simulink model "EGRVlv_VDMon"  (R2018a)
settings: configuration reference "cs_ert" (kept outside this file)
model workspace (MAT data in the model file):
  EGRVlv_VDMon_DT = 10
values from neighbouring files (symbols this model uses):
  EGRVlv_drActDvt_C = 2.0    [EGRVlv_VDMon.sldd]
  EGRVlv_drActDvtHi_C = 4.0    [EGRVlv_VDMon.sldd]
  EGRVlv_numJamVlv_C = 2.0    [EGRVlv_VDMon.sldd]
  EGRVlv_numLckdDetThres_C = 0.0    [EGRVlv_VDMon.sldd]
  EGRVlv_numMonEngTemp_C = 0.0    [EGRVlv_VDMon.sldd]
  EGRVlv_rDvtMax_C = 10.0    [EGRVlv_VDMon.sldd]
  EGRVlv_rDvtMin_C = 5.0    [EGRVlv_VDMon.sldd]
  EGRVlv_rLckdDetThres_C = 5.0    [EGRVlv_VDMon.sldd]
  EGRVlv_rLMSActPosThresInit_C = 3.0    [EGRVlv_VDMon.sldd]
  EGRVlv_rLMSActThresDwn_C = 5.0    [EGRVlv_VDMon.sldd]
  EGRVlv_rLMSThresDwn_C = 5.0    [EGRVlv_VDMon.sldd]
  EGRVlv_rLMSThresUp_C = 10.0    [EGRVlv_VDMon.sldd]
  EGRVlv_RlsIKi_C = 5.0    [EGRVlv_VDMon.sldd]
  EGRVlv_rRlsMax_C = 80.0    [EGRVlv_VDMon.sldd]
  EGRVlv_rStpThres_C = 2.0    [EGRVlv_VDMon.sldd]
  EGRVlv_tEngHi_C = 200.0    [EGRVlv_VDMon.sldd]
  EGRVlv_tEngLo_C = 150.0    [EGRVlv_VDMon.sldd]
  EGRVlv_tiGovDvtMaxDebDef_C = 200.0    [EGRVlv_VDMon.sldd]
  EGRVlv_tiGovDvtMaxDebOk_C = 200.0    [EGRVlv_VDMon.sldd]
  EGRVlv_tiGovDvtMinDebDef_C = 200.0    [EGRVlv_VDMon.sldd]
  EGRVlv_tiGovDvtMinDebOk_C = 200.0    [EGRVlv_VDMon.sldd]
  EGRVlv_tiLMS_C = 1.0    [EGRVlv_VDMon.sldd]
  EGRVlv_tiRepRls_C = 1.0    [EGRVlv_VDMon.sldd]
  EGRVlv_tiRls_C = 1.0    [EGRVlv_VDMon.sldd]
undefined symbols (not defined in the file or in its folder): EngState
libraries: simulink x25, sllib x6
settings Model: DataDictionary=EGRVlv_VDMon.sldd  Creator=zhoutinglin  LastModifiedBy=zhoutinglin

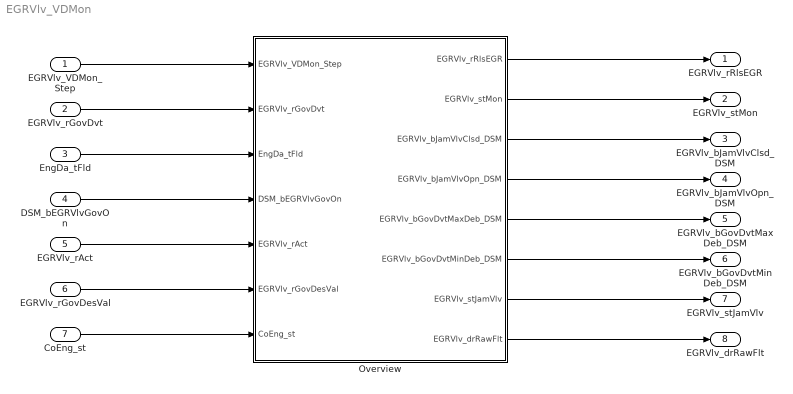
== system EGRVlv_VDMon ==
  EGRVlv_VDMon_Step : Inport  OutputFunctionCall=on
  EGRVlv_rGovDvt : Inport  Description=Control deviation  Port=2  OutMin=-100  OutMax=100  OutDataTypeStr=DutyCycle  Unit=%  PortDimensions=[1 1]
  EngDa_tFld : Inport  Description=Engine temperature field  Port=3  OutMin=-3000  OutMax=3000  OutDataTypeStr=Temp_C  Unit=deg  PortDimensions=[1 3]
  DSM_bEGRVlvGovOn : Inport  Description=Status of FId_EGRVlvGovOn  Port=4  OutMin=0  OutMax=1  OutDataTypeStr=boolean  PortDimensions=[1 1]
  EGRVlv_rAct : Inport  Description=Actuatorposition  Port=5  OutMin=-100  OutMax=100  OutDataTypeStr=DutyCycle  Unit=%  PortDimensions=[1 1]
  EGRVlv_rGovDesVal : Inport  Description=Internal desired value for governor  Port=6  OutMin=-100  OutMax=100  OutDataTypeStr=DutyCycle  Unit=%  PortDimensions=[1 1]
  CoEng_st : Inport  Description=Engine coordinator state  Port=7  OutDataTypeStr=Enum:EngState  PortDimensions=[1 1]
  Overview : Subsystem
  EGRVlv_rRlsEGR : Outport  Description=Additional control value to release a jammed valve  OutMin=-100  OutMax=100  OutDataTypeStr=DutyCycle  Unit=%  PortDimensions=[1 1]
  EGRVlv_stMon : Outport  Description=State of system monitoring  Port=2  OutMin=0  OutMax=65535  OutDataTypeStr=State2  PortDimensions=[1 1]
  EGRVlv_bJamVlvClsd_DSM : Outport  Description=Status of EGRVlv_bJamVlvClsd  Port=3  OutMin=0  OutMax=1  OutDataTypeStr=boolean  PortDimensions=[1 1]
  EGRVlv_bJamVlvOpn_DSM : Outport  Description=Status of EGRVlv_bJamVlvOpn  Port=4  OutMin=0  OutMax=1  OutDataTypeStr=boolean  PortDimensions=[1 1]
  EGRVlv_bGovDvtMaxDeb_DSM : Outport  Description=Status of EGRVlv_bGovDvtMaxDeb  Port=5  OutMin=0  OutMax=1  OutDataTypeStr=boolean  PortDimensions=[1 1]
  EGRVlv_bGovDvtMinDeb_DSM : Outport  Description=Status of EGRVlv_bGovDvtMinDeb  Port=6  OutMin=0  OutMax=1  OutDataTypeStr=boolean  PortDimensions=[1 1]
  EGRVlv_stJamVlv : Outport  Description=Status indicates that the valve is jammed  Port=7  OutMin=0  OutMax=1  OutDataTypeStr=boolean  PortDimensions=[1 1]
  EGRVlv_drRawFlt : Outport  Description=EGR rate gradient calculated over current position after PT1-filtering  Port=8  OutMin=-100  OutMax=100  OutDataTypeStr=DutyCycle  Unit=r/s  PortDimensions=[1 1]
  wires:
  EGRVlv_VDMon_Step/1 -> Overview/1(EGRVlv_VDMon_Step)
  EGRVlv_rGovDvt/1 -> Overview/2(EGRVlv_rGovDvt)
  EngDa_tFld/1 -> Overview/3(EngDa_tFld)
  DSM_bEGRVlvGovOn/1 -> Overview/4(DSM_bEGRVlvGovOn)
  EGRVlv_rAct/1 -> Overview/5(EGRVlv_rAct)
  EGRVlv_rGovDesVal/1 -> Overview/6(EGRVlv_rGovDesVal)
  CoEng_st/1 -> Overview/7(CoEng_st)
  Overview/1(EGRVlv_rRlsEGR) -> EGRVlv_rRlsEGR/1
  Overview/2(EGRVlv_stMon) -> EGRVlv_stMon/1
  Overview/3(EGRVlv_bJamVlvClsd_DSM) -> EGRVlv_bJamVlvClsd_DSM/1
  Overview/4(EGRVlv_bJamVlvOpn_DSM) -> EGRVlv_bJamVlvOpn_DSM/1
  Overview/5(EGRVlv_bGovDvtMaxDeb_DSM) -> EGRVlv_bGovDvtMaxDeb_DSM/1
  Overview/6(EGRVlv_bGovDvtMinDeb_DSM) -> EGRVlv_bGovDvtMinDeb_DSM/1
  Overview/7(EGRVlv_stJamVlv) -> EGRVlv_stJamVlv/1
  Overview/8(EGRVlv_drRawFlt) -> EGRVlv_drRawFlt/1

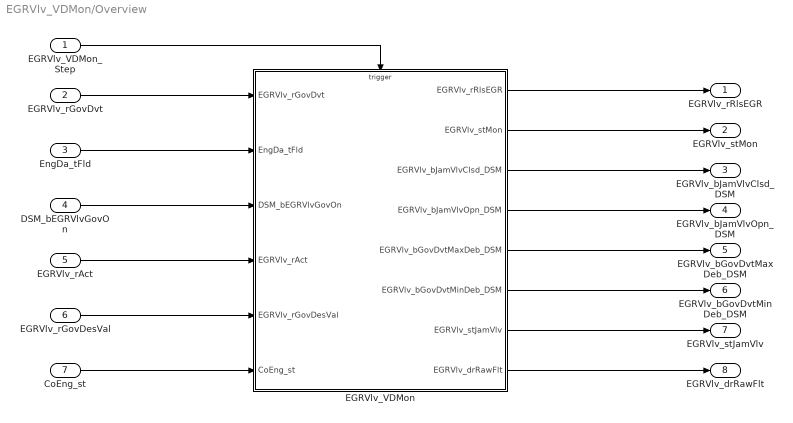
== system EGRVlv_VDMon/Overview ==
  EGRVlv_VDMon_Step : Inport
  EGRVlv_rGovDvt : Inport  Port=2
  EngDa_tFld : Inport  Port=3
  DSM_bEGRVlvGovOn : Inport  Port=4
  EGRVlv_rAct : Inport  Port=5
  EGRVlv_rGovDesVal : Inport  Port=6
  CoEng_st : Inport  Port=7
  EGRVlv_VDMon : Subsystem
  EGRVlv_rRlsEGR : Outport
  EGRVlv_stMon : Outport  Port=2
  EGRVlv_bJamVlvClsd_DSM : Outport  Port=3
  EGRVlv_bJamVlvOpn_DSM : Outport  Port=4
  EGRVlv_bGovDvtMaxDeb_DSM : Outport  Port=5
  EGRVlv_bGovDvtMinDeb_DSM : Outport  Port=6
  EGRVlv_stJamVlv : Outport  Port=7
  EGRVlv_drRawFlt : Outport  Port=8
  wires:
  EGRVlv_rGovDvt/1 -> EGRVlv_VDMon/1(EGRVlv_rGovDvt)
  EngDa_tFld/1 -> EGRVlv_VDMon/2(EngDa_tFld)
  DSM_bEGRVlvGovOn/1 -> EGRVlv_VDMon/3(DSM_bEGRVlvGovOn)
  EGRVlv_rAct/1 -> EGRVlv_VDMon/4(EGRVlv_rAct)
  EGRVlv_rGovDesVal/1 -> EGRVlv_VDMon/5(EGRVlv_rGovDesVal)
  CoEng_st/1 -> EGRVlv_VDMon/6(CoEng_st)
  EGRVlv_VDMon/1(EGRVlv_rRlsEGR) -> EGRVlv_rRlsEGR/1
  EGRVlv_VDMon/2(EGRVlv_stMon) -> EGRVlv_stMon/1
  EGRVlv_VDMon/3(EGRVlv_bJamVlvClsd_DSM) -> EGRVlv_bJamVlvClsd_DSM/1
  EGRVlv_VDMon/4(EGRVlv_bJamVlvOpn_DSM) -> EGRVlv_bJamVlvOpn_DSM/1
  EGRVlv_VDMon/5(EGRVlv_bGovDvtMaxDeb_DSM) -> EGRVlv_bGovDvtMaxDeb_DSM/1
  EGRVlv_VDMon/6(EGRVlv_bGovDvtMinDeb_DSM) -> EGRVlv_bGovDvtMinDeb_DSM/1
  EGRVlv_VDMon/7(EGRVlv_stJamVlv) -> EGRVlv_stJamVlv/1
  EGRVlv_VDMon/8(EGRVlv_drRawFlt) -> EGRVlv_drRawFlt/1
  EGRVlv_VDMon_Step/1 -> EGRVlv_VDMon/Trigger

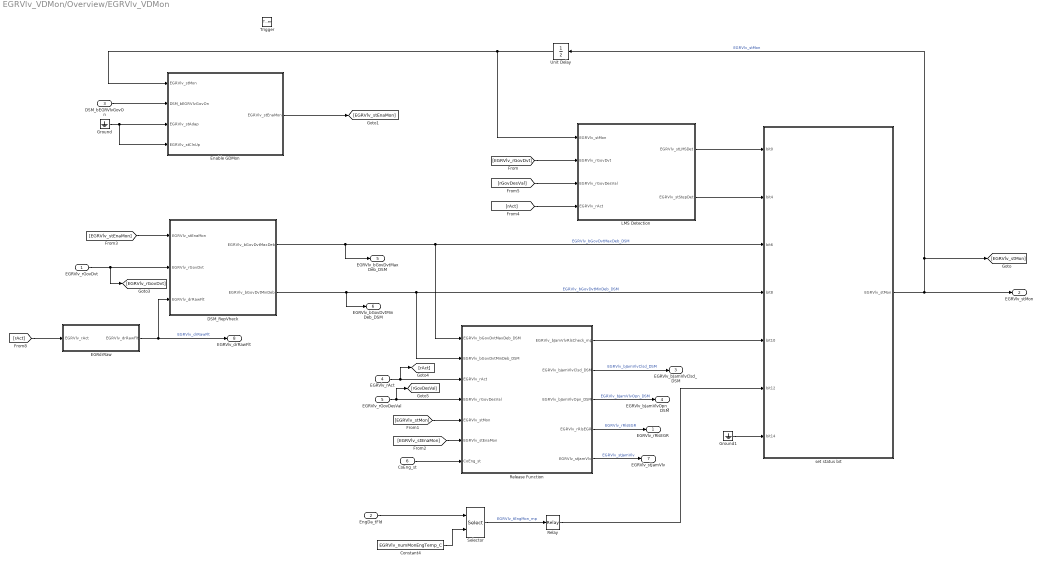
== system EGRVlv_VDMon/Overview/EGRVlv_VDMon ==
  EGRVlv_rGovDvt : Inport  Tag=%
  EngDa_tFld : Inport  Tag=%  Port=2
  DSM_bEGRVlvGovOn : Inport  Tag=%  Port=3
  EGRVlv_rAct : Inport  Tag=%  Port=4
  EGRVlv_rGovDesVal : Inport  Tag=%  Port=5
  CoEng_st : Inport  Tag=%  Port=6
  Trigger : TriggerPort  TriggerType=function-call  VariantControl=Variant  PortDimensions=1
  Constant4 : Constant  Value=EGRVlv_numMonEngTemp_C  SampleTime=-1
  DSM_RepVheck : Subsystem
  EGRdrRaw : Subsystem
  Enable GDMon : Subsystem
  Ground : Ground
  Ground1 : Ground
  LMS Detection : Subsystem
  Relay : Relay  OnSwitchValue=EGRVlv_tEngHi_C  OffSwitchValue=EGRVlv_tEngLo_C
  Release Function : Subsystem
  Selector : Selector  IndexMode=Zero-based  InputPortWidth=3  IndexOptions=Index vector (port)  Indices=[1 3]  OutputSizes=1
  Unit Delay : UnitDelay  SampleTime=-1
      settings: AttributesFormatString=InitialValue=%<InitialCondition>
  set status bit : Subsystem
  EGRVlv_rRlsEGR : Outport  Tag=%
  EGRVlv_stMon : Outport  Tag=%  Port=2
  EGRVlv_bJamVlvClsd_DSM : Outport  Tag=%  Port=3
  EGRVlv_bJamVlvOpn_DSM : Outport  Tag=%  Port=4
  EGRVlv_bGovDvtMaxDeb_DSM : Outport  Port=5
  EGRVlv_bGovDvtMinDeb_DSM : Outport  Port=6
  EGRVlv_stJamVlv : Outport  Port=7
  EGRVlv_drRawFlt : Outport  Port=8
  wires:
  Selector/1 -> Relay/1  "EGRVlv_tEngMon_mp"
  set status bit/1(EGRVlv_stMon) -> EGRVlv_stMon/1, Unit Delay/1, [EGRVlv_stMon]  "EGRVlv_stMon"
  Constant4/1 -> Selector/2
  EngDa_tFld/1 -> Selector/1
  EGRVlv_rGovDvt/1 -> [EGRVlv_rGovDvt], DSM_RepVheck/2(EGRVlv_rGovDvt)
  EGRVlv_rAct/1 -> [rAct], Release Function/3(EGRVlv_rAct)
  EGRVlv_rGovDesVal/1 -> [rGovDesVal], Release Function/4(EGRVlv_rGovDesVal)
  Unit Delay/1 -> Enable GDMon/1(EGRVlv_stMon), LMS Detection/1(EGRVlv_stMon)
  LMS Detection/2(EGRVlv_stStepDet) -> set status bit/2(bit4)
  LMS Detection/1(EGRVlv_stLMSDet) -> set status bit/1(bit0)
  Enable GDMon/1(EGRVlv_stEnaMon) -> [EGRVlv_stEnaMon]
  DSM_bEGRVlvGovOn/1 -> Enable GDMon/2(DSM_bEGRVlvGovOn)
  Ground/1 -> Enable GDMon/4(EGRVlv_stClnUp), Enable GDMon/3(EGRVlv_stAdap)
  [EGRVlv_rGovDvt] -> LMS Detection/2(EGRVlv_rGovDvt)
  [rGovDesVal] -> LMS Detection/3(EGRVlv_rGovDesVal)
  [rAct] -> LMS Detection/4(EGRVlv_rAct)
  [EGRVlv_stMon] -> Release Function/5(EGRVlv_stMon)
  [EGRVlv_stEnaMon] -> Release Function/6(EGRVlv_stEnaMon)
  CoEng_st/1 -> Release Function/7(CoEng_st)
  Ground1/1 -> set status bit/7(bit14)
  Release Function/2(EGRVlv_bJamVlvClsd_DSM) -> EGRVlv_bJamVlvClsd_DSM/1  "EGRVlv_bJamVlvClsd_DSM"
  Release Function/3(EGRVlv_bJamVlvOpn_DSM) -> EGRVlv_bJamVlvOpn_DSM/1  "EGRVlv_bJamVlvOpn_DSM"
  Release Function/4(EGRVlv_rRlsEGR) -> EGRVlv_rRlsEGR/1  "EGRVlv_rRlsEGR"
  DSM_RepVheck/2(EGRVlv_bGovDvtMinDeb) -> Release Function/2(EGRVlv_bGovDvtMinDeb_DSM), set status bit/4(bit8), EGRVlv_bGovDvtMinDeb_DSM/1  "EGRVlv_bGovDvtMinDeb_DSM"
  DSM_RepVheck/1(EGRVlv_bGovDvtMaxDeb) -> set status bit/3(bit6), Release Function/1(EGRVlv_bGovDvtMaxDeb_DSM), EGRVlv_bGovDvtMaxDeb_DSM/1  "EGRVlv_bGovDvtMaxDeb_DSM"
  Relay/1 -> set status bit/6(bit12)
  Release Function/1(EGRVlv_bJamVlvRlsCheck_mp) -> set status bit/5(bit10)
  Release Function/5(EGRVlv_stJamVlv) -> EGRVlv_stJamVlv/1  "EGRVlv_stJamVlv"
  [rAct] -> EGRdrRaw/1(EGRVlv_rAct)
  EGRdrRaw/1(EGRVlv_drRawFlt) -> DSM_RepVheck/3(EGRVlv_drRawFlt), EGRVlv_drRawFlt/1  "EGRVlv_drRawFlt"
  [EGRVlv_stEnaMon] -> DSM_RepVheck/1(EGRVlv_stEnaMon)

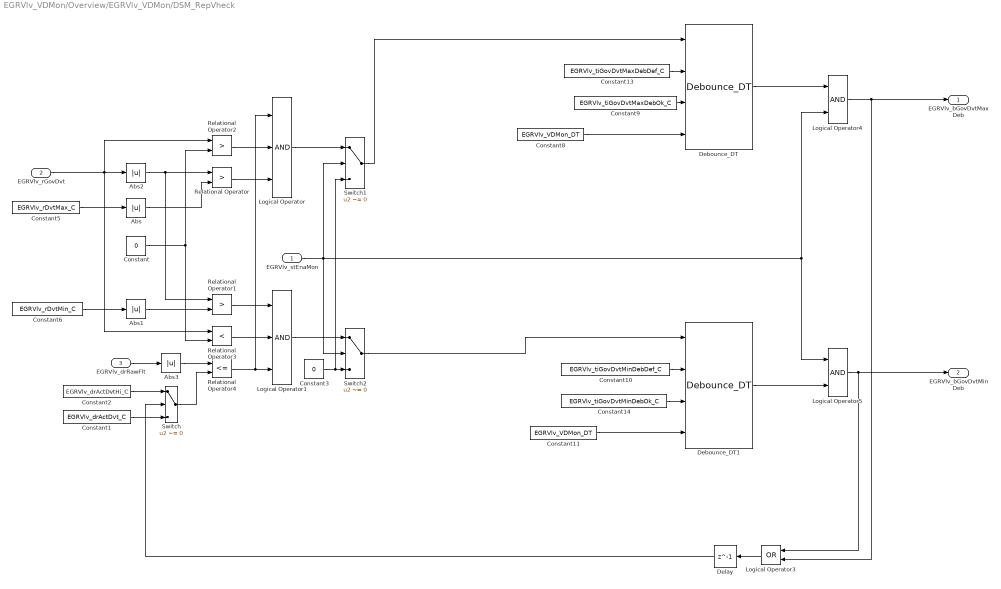
== system EGRVlv_VDMon/Overview/EGRVlv_VDMon/DSM_RepVheck ==
  EGRVlv_stEnaMon : Inport
  EGRVlv_rGovDvt : Inport  Tag=%  Port=2
  EGRVlv_drRawFlt : Inport  Port=3
  Abs{,1..3} (4 alike) : Abs
  Constant : Constant  Value=0  OutDataTypeStr=Inherit: Inherit via back propagation
  Constant1 : Constant  Value=EGRVlv_drActDvt_C  SampleTime=-1
  Constant10 : Constant  Value=EGRVlv_tiGovDvtMinDebDef_C
  Constant11 : Constant  Value=EGRVlv_VDMon_DT  OutDataTypeStr=Inherit: Inherit via back propagation
  Constant13 : Constant  Value=EGRVlv_tiGovDvtMaxDebDef_C
  Constant14 : Constant  Value=EGRVlv_tiGovDvtMinDebOk_C
  Constant2 : Constant  Value=EGRVlv_drActDvtHi_C  SampleTime=-1
  Constant3 : Constant  Value=0  OutDataTypeStr=Inherit: Inherit via back propagation
  Constant5 : Constant  Value=EGRVlv_rDvtMax_C  SampleTime=-1
  Constant6 : Constant  Value=EGRVlv_rDvtMin_C  SampleTime=-1
  Constant8 : Constant  Value=EGRVlv_VDMon_DT  OutDataTypeStr=Inherit: Inherit via back propagation
  Constant9 : Constant  Value=EGRVlv_tiGovDvtMaxDebOk_C
  Debounce_DT : sllib/Debounce_DT
      settings: SourceProductName=sllib
  Debounce_DT1 : sllib/Debounce_DT
      settings: SourceProductName=sllib
  Delay : Delay  DelayLength=1  InitialCondition=0
  Logical Operator : Logic  Inputs=3  AllPortsSameDT=off  OutDataTypeStr=boolean
  Logical Operator1 : Logic  Inputs=3  AllPortsSameDT=off  OutDataTypeStr=boolean
  Logical Operator3 : Logic  Operator=OR  AllPortsSameDT=off  OutDataTypeStr=boolean
  Logical Operator4 : Logic  AllPortsSameDT=off  OutDataTypeStr=boolean
  Logical Operator5 : Logic  AllPortsSameDT=off  OutDataTypeStr=boolean
  Relational Operator : RelationalOperator  Operator=>  OutDataTypeStr=boolean  RndMeth=Simplest  InputSameDT=on
  Relational Operator1 : RelationalOperator  Operator=>  OutDataTypeStr=boolean  RndMeth=Simplest
  Relational Operator2 : RelationalOperator  Operator=>  OutDataTypeStr=boolean  RndMeth=Simplest  InputSameDT=on
  Relational Operator3 : RelationalOperator  Operator=<  OutDataTypeStr=boolean  RndMeth=Simplest
  Relational Operator4 : RelationalOperator  Operator=<=  OutDataTypeStr=boolean  RndMeth=Simplest
  Switch : Switch  Criteria=u2 ~= 0
  Switch1 : Switch  Criteria=u2 ~= 0
  Switch2 : Switch  Criteria=u2 ~= 0
  EGRVlv_bGovDvtMaxDeb : Outport  OutputWhenDisabled=reset  InitialOutput=0
  EGRVlv_bGovDvtMinDeb : Outport  Port=2  OutputWhenDisabled=reset  InitialOutput=0
  wires:
  Relational Operator1/1 -> Logical Operator1/1
  Constant5/1 -> Abs/1
  Relational Operator3/1 -> Logical Operator1/2
  Constant8/1 -> Debounce_DT/4
  Abs/1 -> Relational Operator/2
  Abs2/1 -> Relational Operator1/1, Relational Operator/1
  Abs3/1 -> Relational Operator4/1
  EGRVlv_drRawFlt/1 -> Abs3/1
  Constant11/1 -> Debounce_DT1/4
  EGRVlv_rGovDvt/1 -> Relational Operator3/1, Relational Operator2/1, Abs2/1
  Constant13/1 -> Debounce_DT/2
  Relational Operator4/1 -> Logical Operator/1, Logical Operator1/3
  Relational Operator/1 -> Logical Operator/3
  Relational Operator2/1 -> Logical Operator/2
  Constant/1 -> Relational Operator3/2, Relational Operator2/2
  Abs1/1 -> Relational Operator1/2
  Constant14/1 -> Debounce_DT1/3
  Constant6/1 -> Abs1/1
  Constant10/1 -> Debounce_DT1/2
  Logical Operator3/1 -> Delay/1
  Delay/1 -> Switch/2
  Constant1/1 -> Switch/3
  Constant2/1 -> Switch/1
  Switch/1 -> Relational Operator4/2
  Switch1/1 -> Debounce_DT/1
  Logical Operator/1 -> Switch1/1
  Switch2/1 -> Debounce_DT1/1
  Logical Operator1/1 -> Switch2/1
  EGRVlv_stEnaMon/1 -> Switch1/2, Logical Operator5/1, Logical Operator4/2, Switch2/2
  Constant3/1 -> Switch1/3, Switch2/3
  Logical Operator4/1 -> EGRVlv_bGovDvtMaxDeb/1, Logical Operator3/2
  Debounce_DT/1 -> Logical Operator4/1
  Logical Operator5/1 -> EGRVlv_bGovDvtMinDeb/1, Logical Operator3/1
  Debounce_DT1/1 -> Logical Operator5/2
  Constant9/1 -> Debounce_DT/3

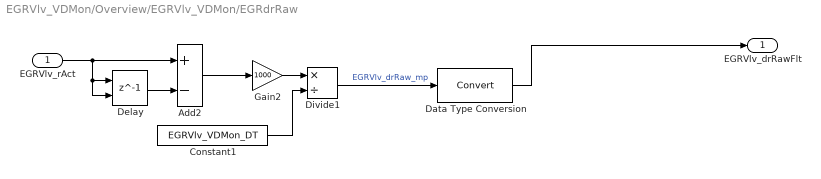
== system EGRVlv_VDMon/Overview/EGRVlv_VDMon/EGRdrRaw ==
  EGRVlv_rAct : Inport
  Add2 : Sum  Inputs=+-  SaturateOnIntegerOverflow=on
  Constant1 : Constant  Value=EGRVlv_VDMon_DT
  Data Type Conversion : DataTypeConversion
  Delay : Delay  DelayLength=1  InitialConditionSource=Input port  InitialCondition=0
      settings: InputPortMap=u0,p4
  Divide1 : Product  Inputs=*/  OutDataTypeStr=Inherit: Inherit via back propagation
  Gain2 : Gain  Gain=1000  OutDataTypeStr=fixdt(1,32,0.0001,0)  SaturateOnIntegerOverflow=on
  EGRVlv_drRawFlt : Outport
  wires:
  Delay/1 -> Add2/2
  EGRVlv_rAct/1 -> Delay/2, Delay/1, Add2/1
  Constant1/1 -> Divide1/2
  Gain2/1 -> Divide1/1
  Add2/1 -> Gain2/1
  Divide1/1 -> Data Type Conversion/1  "EGRVlv_drRaw_mp"
  Data Type Conversion/1 -> EGRVlv_drRawFlt/1

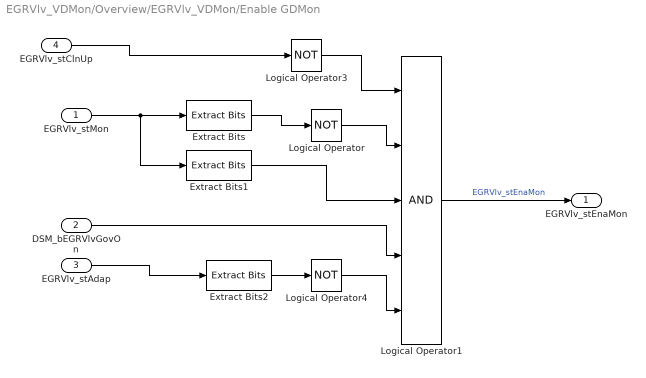
== system EGRVlv_VDMon/Overview/EGRVlv_VDMon/Enable GDMon ==
  EGRVlv_stMon : Inport  Tag=%
  DSM_bEGRVlvGovOn : Inport  Tag=%  Port=2
  EGRVlv_stAdap : Inport  Tag=%  Port=3
  EGRVlv_stClnUp : Inport  Tag=%  Port=4
  Extract Bits : simulink/Logic and Bit Operations/Extract Bits  bitsToExtract=Range of bits  numBits=8  bitIdxRange=[10 10]  outScalingMode=Treat bit field as an integer
      settings: SourceProductName=Simulink
  Extract Bits1 : simulink/Logic and Bit Operations/Extract Bits  bitsToExtract=Range of bits  numBits=8  bitIdxRange=[12 12]  outScalingMode=Treat bit field as an integer
      settings: SourceProductName=Simulink
  Extract Bits2 : simulink/Logic and Bit Operations/Extract Bits  bitsToExtract=Range of bits  numBits=8  bitIdxRange=[0 0]  outScalingMode=Treat bit field as an integer
      settings: SourceProductName=Simulink
  Logical Operator : Logic  Operator=NOT  AllPortsSameDT=off  OutDataTypeStr=boolean
  Logical Operator1 : Logic  Inputs=5  AllPortsSameDT=off  OutDataTypeStr=boolean
  Logical Operator3 : Logic  Operator=NOT  AllPortsSameDT=off  OutDataTypeStr=boolean
  Logical Operator4 : Logic  Operator=NOT  AllPortsSameDT=off  OutDataTypeStr=boolean
  EGRVlv_stEnaMon : Outport  Tag=%
  wires:
  Logical Operator/1 -> Logical Operator1/2
  Extract Bits1/1 -> Logical Operator1/3
  Extract Bits2/1 -> Logical Operator4/1
  EGRVlv_stClnUp/1 -> Logical Operator3/1
  Logical Operator4/1 -> Logical Operator1/5
  Logical Operator1/1 -> EGRVlv_stEnaMon/1  "EGRVlv_stEnaMon"
  DSM_bEGRVlvGovOn/1 -> Logical Operator1/4
  Extract Bits/1 -> Logical Operator/1
  EGRVlv_stMon/1 -> Extract Bits1/1, Extract Bits/1
  EGRVlv_stAdap/1 -> Extract Bits2/1
  Logical Operator3/1 -> Logical Operator1/1

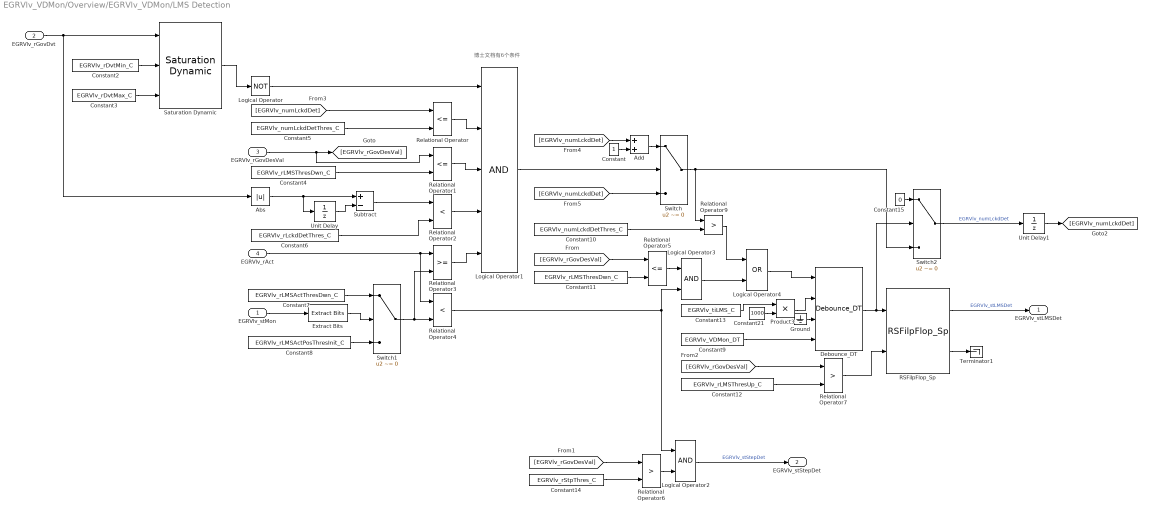
== system EGRVlv_VDMon/Overview/EGRVlv_VDMon/LMS Detection ==
  note: 博士文档有6个条件
  EGRVlv_stMon : Inport  Tag=%
  EGRVlv_rGovDvt : Inport  Tag=%  Port=2
  EGRVlv_rGovDesVal : Inport  Tag=%  Port=3
  EGRVlv_rAct : Inport  Tag=%  Port=4
  Abs : Abs
  Add : Sum  SaturateOnIntegerOverflow=on
  Constant : Constant  OutDataTypeStr=Inherit: Inherit via back propagation
  Constant10 : Constant  Value=EGRVlv_numLckdDetThres_C
  Constant11 : Constant  Value=EGRVlv_rLMSThresDwn_C
  Constant12 : Constant  Value=EGRVlv_rLMSThresUp_C
  Constant13 : Constant  Value=EGRVlv_tiLMS_C
  Constant14 : Constant  Value=EGRVlv_rStpThres_C
  Constant15 : Constant  Value=0  OutDataTypeStr=Inherit: Inherit via back propagation
  Constant2 : Constant  Value=EGRVlv_rDvtMin_C  SampleTime=-1
  Constant21 : Constant  Value=1000  OutDataTypeStr=uint16
  Constant3 : Constant  Value=EGRVlv_rDvtMax_C  SampleTime=-1
  Constant4 : Constant  Value=EGRVlv_rLMSThresDwn_C  SampleTime=-1
  Constant5 : Constant  Value=EGRVlv_numLckdDetThres_C  SampleTime=-1
  Constant6 : Constant  Value=EGRVlv_rLckdDetThres_C  SampleTime=-1
  Constant7 : Constant  Value=EGRVlv_rLMSActThresDwn_C  SampleTime=-1
  Constant8 : Constant  Value=EGRVlv_rLMSActPosThresInit_C  SampleTime=-1
  Constant9 : Constant  Value=EGRVlv_VDMon_DT
  Debounce_DT : sllib/Debounce_DT
      settings: SourceProductName=sllib
  Extract Bits : simulink/Logic and Bit Operations/Extract Bits  bitsToExtract=Range of bits  numBits=8  bitIdxRange=[14 14]  outScalingMode=Treat bit field as an integer
      settings: SourceProductName=Simulink
  Ground : Ground
  Logical Operator : Logic  Operator=NOT  AllPortsSameDT=off  OutDataTypeStr=boolean
  Logical Operator1 : Logic  Inputs=5  AllPortsSameDT=off  OutDataTypeStr=boolean
  Logical Operator2 : Logic  AllPortsSameDT=off  OutDataTypeStr=boolean
  Logical Operator3 : Logic  AllPortsSameDT=off  OutDataTypeStr=boolean
  Logical Operator4 : Logic  Operator=OR  AllPortsSameDT=off  OutDataTypeStr=boolean
  Product3 : Product  OutDataTypeStr=uint32  SaturateOnIntegerOverflow=on
  RSFilpFlop_Sp : sllib/RSFilpFlop_Sp
      settings: SourceProductName=sllib
  Relational Operator : RelationalOperator  Operator=<=  OutDataTypeStr=boolean  RndMeth=Simplest
  Relational Operator1 : RelationalOperator  Operator=<=  OutDataTypeStr=boolean  RndMeth=Simplest
  Relational Operator2 : RelationalOperator  Operator=<  OutDataTypeStr=boolean  RndMeth=Simplest
  Relational Operator3 : RelationalOperator  OutDataTypeStr=boolean  RndMeth=Simplest
  Relational Operator4 : RelationalOperator  Operator=<  OutDataTypeStr=boolean  RndMeth=Simplest
  Relational Operator5 : RelationalOperator  Operator=<=  OutDataTypeStr=boolean  RndMeth=Simplest
  Relational Operator6 : RelationalOperator  Operator=>  OutDataTypeStr=boolean  RndMeth=Simplest
  Relational Operator7 : RelationalOperator  Operator=>  OutDataTypeStr=boolean  RndMeth=Simplest
  Relational Operator9 : RelationalOperator  Operator=>  OutDataTypeStr=boolean  RndMeth=Simplest
  Saturation Dynamic : simulink/Discontinuities/Saturation Dynamic  OutMin=[]  OutMax=[]  OutDataTypeStr=Inherit: Same as second input  OutDataType=fixdt(1, 16)  OutScaling=2^-10  DoSatur=off
  Subtract : Sum  Inputs=+-  SaturateOnIntegerOverflow=on
  Switch : Switch  Criteria=u2 ~= 0
  Switch1 : Switch  Criteria=u2 ~= 0
  Switch2 : Switch  Criteria=u2 ~= 0
  Terminator1 : Terminator
  Unit Delay : UnitDelay  SampleTime=-1
      settings: AttributesFormatString=InitialValue=%<InitialCondition>
  Unit Delay1 : UnitDelay  SampleTime=-1
      settings: AttributesFormatString=InitialValue=%<InitialCondition>
  EGRVlv_stLMSDet : Outport  Tag=%
  EGRVlv_stStepDet : Outport  Tag=%  Port=2
  wires:
  Saturation Dynamic/1 -> Logical Operator/1
  Relational Operator/1 -> Logical Operator1/2
  Relational Operator1/1 -> Logical Operator1/3
  Relational Operator2/1 -> Logical Operator1/4
  Relational Operator3/1 -> Logical Operator1/5
  Constant5/1 -> Relational Operator/2
  Constant2/1 -> Saturation Dynamic/2
  Constant3/1 -> Saturation Dynamic/3
  EGRVlv_rGovDvt/1 -> Saturation Dynamic/1, Abs/1
  [EGRVlv_numLckdDet] -> Relational Operator/1
  Constant4/1 -> Relational Operator1/2
  EGRVlv_rGovDesVal/1 -> [EGRVlv_rGovDesVal], Relational Operator1/1
  Subtract/1 -> Relational Operator2/1
  Abs/1 -> Unit Delay/1, Subtract/1
  Unit Delay/1 -> Subtract/2
  Constant6/1 -> Relational Operator2/2
  Logical Operator1/1 -> Switch/2
  Add/1 -> Switch/1
  Constant/1 -> Add/2
  Constant7/1 -> Switch1/1
  Constant8/1 -> Switch1/3
  Extract Bits/1 -> Switch1/2
  Switch1/1 -> Relational Operator3/2, Relational Operator4/2
  Relational Operator6/1 -> Logical Operator2/2
  Relational Operator4/1 -> Logical Operator2/1, Logical Operator3/2
  Relational Operator5/1 -> Logical Operator3/1
  Logical Operator3/1 -> Logical Operator4/2
  Relational Operator9/1 -> Logical Operator4/1
  Constant9/1 -> Debounce_DT/4
  Debounce_DT/1 -> RSFilpFlop_Sp/1, Switch2/2
  Logical Operator4/1 -> Debounce_DT/1
  Relational Operator7/1 -> RSFilpFlop_Sp/2
  Constant10/1 -> Relational Operator9/2
  [EGRVlv_rGovDesVal] -> Relational Operator5/1
  Constant11/1 -> Relational Operator5/2
  Constant12/1 -> Relational Operator7/2
  Constant14/1 -> Relational Operator6/2
  [EGRVlv_rGovDesVal] -> Relational Operator7/1
  Logical Operator2/1 -> EGRVlv_stStepDet/1  "EGRVlv_stStepDet"
  EGRVlv_rAct/1 -> Relational Operator4/1, Relational Operator3/1
  Constant15/1 -> Switch2/1
  Switch2/1 -> Unit Delay1/1  "EGRVlv_numLckdDet"
  Unit Delay1/1 -> [EGRVlv_numLckdDet]
  [EGRVlv_numLckdDet] -> Add/1
  [EGRVlv_numLckdDet] -> Switch/3
  Switch/1 -> Relational Operator9/1, Switch2/3
  [EGRVlv_rGovDesVal] -> Relational Operator6/1
  Logical Operator/1 -> Logical Operator1/1
  Constant21/1 -> Product3/2
  Constant13/1 -> Product3/1
  Product3/1 -> Debounce_DT/2
  EGRVlv_stMon/1 -> Extract Bits/1
  RSFilpFlop_Sp/1 -> EGRVlv_stLMSDet/1  "EGRVlv_stLMSDet"
  RSFilpFlop_Sp/2 -> Terminator1/1
  Ground/1 -> Debounce_DT/3

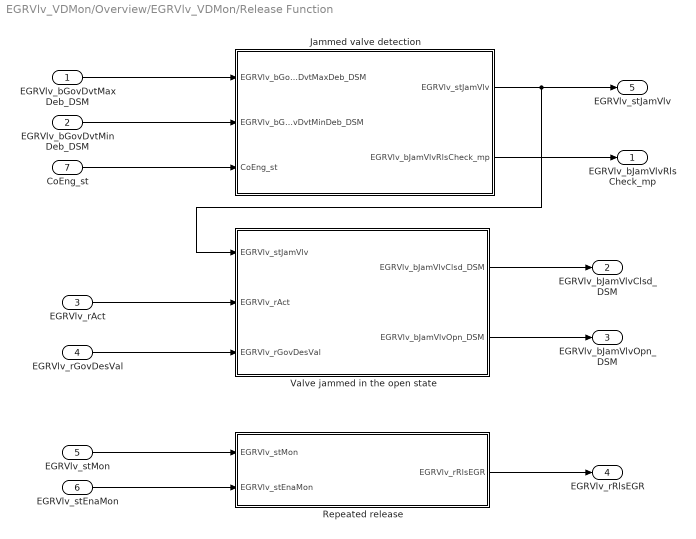
== system EGRVlv_VDMon/Overview/EGRVlv_VDMon/Release Function ==
  EGRVlv_bGovDvtMaxDeb_DSM : Inport  Tag=%
  EGRVlv_bGovDvtMinDeb_DSM : Inport  Tag=%  Port=2
  EGRVlv_rAct : Inport  Tag=%  Port=3
  EGRVlv_rGovDesVal : Inport  Tag=%  Port=4
  EGRVlv_stMon : Inport  Tag=%  Port=5
  EGRVlv_stEnaMon : Inport  Tag=%  Port=6
  CoEng_st : Inport  Tag=%  Port=7
  Jammed valve detection : Subsystem
  Repeated release : Subsystem
  Valve jammed in the open state : Subsystem
  EGRVlv_bJamVlvRlsCheck_mp : Outport
  EGRVlv_bJamVlvClsd_DSM : Outport  Tag=%  Port=2
  EGRVlv_bJamVlvOpn_DSM : Outport  Tag=%  Port=3
  EGRVlv_rRlsEGR : Outport  Tag=%  Port=4
  EGRVlv_stJamVlv : Outport  Tag=%  Port=5
  wires:
  EGRVlv_bGovDvtMinDeb_DSM/1 -> Jammed valve detection/2(EGRVlv_bGovDvtMinDeb_DSM)
  Jammed valve detection/1(EGRVlv_stJamVlv) -> Valve jammed in the open state/1(EGRVlv_stJamVlv), EGRVlv_stJamVlv/1
  EGRVlv_bGovDvtMaxDeb_DSM/1 -> Jammed valve detection/1(EGRVlv_bGovDvtMaxDeb_DSM)
  CoEng_st/1 -> Jammed valve detection/3(CoEng_st)
  EGRVlv_stMon/1 -> Repeated release/1(EGRVlv_stMon)
  EGRVlv_stEnaMon/1 -> Repeated release/2(EGRVlv_stEnaMon)
  EGRVlv_rAct/1 -> Valve jammed in the open state/2(EGRVlv_rAct)
  EGRVlv_rGovDesVal/1 -> Valve jammed in the open state/3(EGRVlv_rGovDesVal)
  Repeated release/1(EGRVlv_rRlsEGR) -> EGRVlv_rRlsEGR/1
  Valve jammed in the open state/1(EGRVlv_bJamVlvClsd_DSM) -> EGRVlv_bJamVlvClsd_DSM/1
  Valve jammed in the open state/2(EGRVlv_bJamVlvOpn_DSM) -> EGRVlv_bJamVlvOpn_DSM/1
  Jammed valve detection/2(EGRVlv_bJamVlvRlsCheck_mp) -> EGRVlv_bJamVlvRlsCheck_mp/1

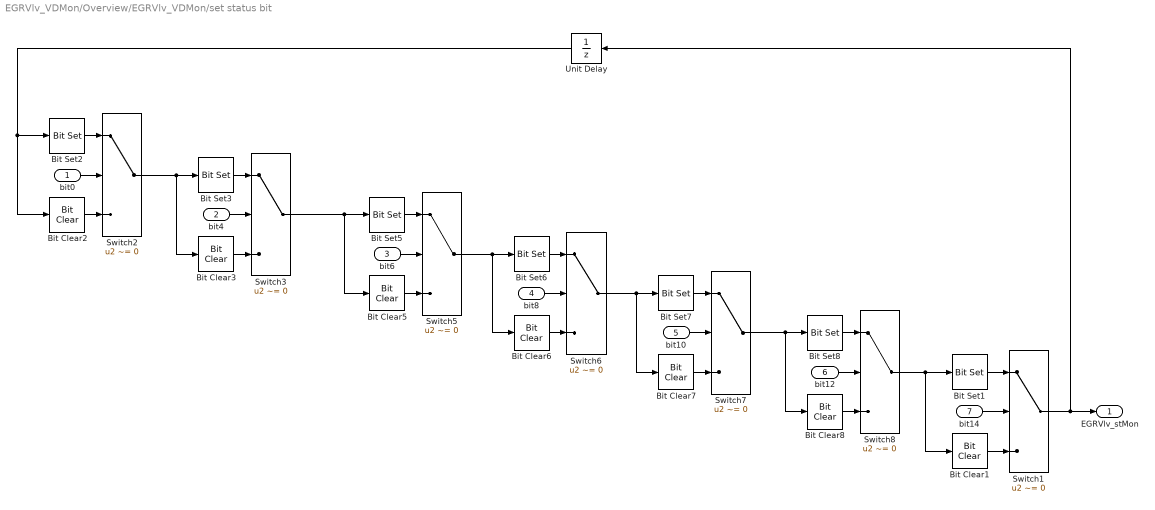
== system EGRVlv_VDMon/Overview/EGRVlv_VDMon/set status bit ==
  bit0 : Inport
  bit4 : Inport  Port=2
  bit6 : Inport  Port=3
  bit8 : Inport  Port=4
  bit10 : Inport  Port=5
  bit12 : Inport  Port=6
  bit14 : Inport  Port=7
  Bit Clear1 : simulink/Logic and Bit Operations/Bit Clear  iBit=14
      settings: SourceProductName=Simulink  SourceProductBaseCode=SL
  Bit Clear2 : simulink/Logic and Bit Operations/Bit Clear  iBit=0
      settings: SourceProductName=Simulink  SourceProductBaseCode=SL
  Bit Clear3 : simulink/Logic and Bit Operations/Bit Clear  iBit=4
      settings: SourceProductName=Simulink  SourceProductBaseCode=SL
  Bit Clear5 : simulink/Logic and Bit Operations/Bit Clear  iBit=6
      settings: SourceProductName=Simulink  SourceProductBaseCode=SL
  Bit Clear6 : simulink/Logic and Bit Operations/Bit Clear  iBit=8
      settings: SourceProductName=Simulink  SourceProductBaseCode=SL
  Bit Clear7 : simulink/Logic and Bit Operations/Bit Clear  iBit=10
      settings: SourceProductName=Simulink  SourceProductBaseCode=SL
  Bit Clear8 : simulink/Logic and Bit Operations/Bit Clear  iBit=12
      settings: SourceProductName=Simulink  SourceProductBaseCode=SL
  Bit Set1 : simulink/Logic and Bit Operations/Bit Set  iBit=14
      settings: SourceProductName=Simulink  SourceProductBaseCode=SL
  Bit Set2 : simulink/Logic and Bit Operations/Bit Set  iBit=0
      settings: SourceProductName=Simulink  SourceProductBaseCode=SL
  Bit Set3 : simulink/Logic and Bit Operations/Bit Set  iBit=4
      settings: SourceProductName=Simulink  SourceProductBaseCode=SL
  Bit Set5 : simulink/Logic and Bit Operations/Bit Set  iBit=6
      settings: SourceProductName=Simulink  SourceProductBaseCode=SL
  Bit Set6 : simulink/Logic and Bit Operations/Bit Set  iBit=8
      settings: SourceProductName=Simulink  SourceProductBaseCode=SL
  Bit Set7 : simulink/Logic and Bit Operations/Bit Set  iBit=10
      settings: SourceProductName=Simulink  SourceProductBaseCode=SL
  Bit Set8 : simulink/Logic and Bit Operations/Bit Set  iBit=12
      settings: SourceProductName=Simulink  SourceProductBaseCode=SL
  Switch{1..3,5..8} (7 alike) : Switch  Criteria=u2 ~= 0  OutDataTypeStr=Inherit: Inherit via back propagation  SaturateOnIntegerOverflow=on  InputSameDT=on
  Unit Delay : UnitDelay  SampleTime=-1
      settings: AttributesFormatString=InitialValue=%<InitialCondition>
  EGRVlv_stMon : Outport
  wires:
  bit12/1 -> Switch8/2
  Switch7/1 -> Bit Clear8/1, Bit Set8/1
  Bit Clear8/1 -> Switch8/3
  Bit Set8/1 -> Switch8/1
  bit10/1 -> Switch7/2
  Switch6/1 -> Bit Set7/1, Bit Clear7/1
  Bit Clear7/1 -> Switch7/3
  Bit Set7/1 -> Switch7/1
  bit8/1 -> Switch6/2
  Switch5/1 -> Bit Clear6/1, Bit Set6/1
  Bit Clear6/1 -> Switch6/3
  Bit Set6/1 -> Switch6/1
  bit6/1 -> Switch5/2
  Bit Clear5/1 -> Switch5/3
  Bit Set5/1 -> Switch5/1
  bit14/1 -> Switch1/2
  Bit Clear1/1 -> Switch1/3
  Bit Set1/1 -> Switch1/1
  Switch1/1 -> Unit Delay/1, EGRVlv_stMon/1
  Switch8/1 -> Bit Clear1/1, Bit Set1/1
  bit4/1 -> Switch3/2
  Switch2/1 -> Bit Set3/1, Bit Clear3/1
  Bit Clear3/1 -> Switch3/3
  Bit Set3/1 -> Switch3/1
  bit0/1 -> Switch2/2
  Bit Clear2/1 -> Switch2/3
  Bit Set2/1 -> Switch2/1
  Switch3/1 -> Bit Clear5/1, Bit Set5/1
  Unit Delay/1 -> Bit Clear2/1, Bit Set2/1

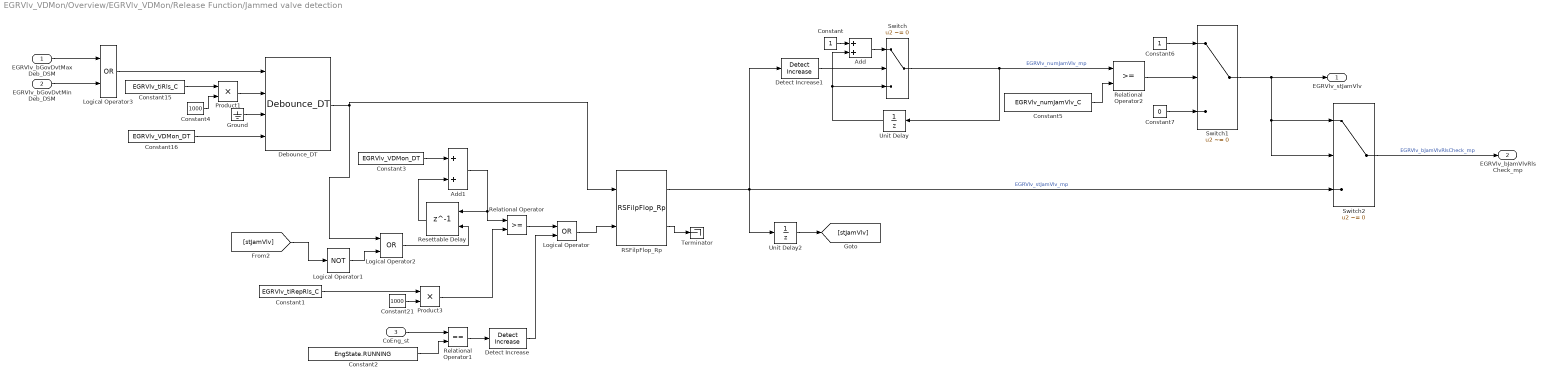
== system EGRVlv_VDMon/Overview/EGRVlv_VDMon/Release Function/Jammed valve detection ==
  EGRVlv_bGovDvtMaxDeb_DSM : Inport  Tag=%
  EGRVlv_bGovDvtMinDeb_DSM : Inport  Tag=%  Port=2
  CoEng_st : Inport  Tag=%  Port=3
  Add : Sum  SaturateOnIntegerOverflow=on
  Add1 : Sum
  Constant : Constant  OutDataTypeStr=uint8
  Constant1 : Constant  Value=EGRVlv_tiRepRls_C
  Constant15 : Constant  Value=EGRVlv_tiRls_C
  Constant16 : Constant  Value=EGRVlv_VDMon_DT
  Constant2 : Constant  Value=EngState.RUNNING
  Constant21 : Constant  Value=1000  OutDataTypeStr=uint16
  Constant3 : Constant  Value=EGRVlv_VDMon_DT
  Constant4 : Constant  Value=1000  OutDataTypeStr=uint16
  Constant5 : Constant  Value=EGRVlv_numJamVlv_C
  Constant6 : Constant  OutDataTypeStr=boolean
  Constant7 : Constant  Value=0  OutDataTypeStr=boolean
  Debounce_DT : sllib/Debounce_DT
      settings: SourceProductName=sllib
  Detect Increase : simulink/Logic and Bit Operations/Detect Increase  vinit=0.0  OutDataTypeStr=boolean
  Detect Increase1 : simulink/Logic and Bit Operations/Detect Increase  vinit=0.0  OutDataTypeStr=boolean
  Ground : Ground
  Logical Operator : Logic  Operator=OR  AllPortsSameDT=off  OutDataTypeStr=boolean
  Logical Operator1 : Logic  Operator=NOT  AllPortsSameDT=off  OutDataTypeStr=boolean
  Logical Operator2 : Logic  Operator=OR  AllPortsSameDT=off  OutDataTypeStr=boolean
  Logical Operator3 : Logic  Operator=OR  AllPortsSameDT=off  OutDataTypeStr=boolean
  Product1 : Product  OutDataTypeStr=uint32  SaturateOnIntegerOverflow=on
  Product3 : Product  OutDataTypeStr=uint32  SaturateOnIntegerOverflow=on
  RSFilpFlop_Rp : sllib/RSFilpFlop_Rp
      settings: SourceProductName=sllib
  Relational Operator : RelationalOperator  OutDataTypeStr=boolean  RndMeth=Simplest
  Relational Operator1 : RelationalOperator  Operator===  OutDataTypeStr=boolean  RndMeth=Simplest
  Relational Operator2 : RelationalOperator  OutDataTypeStr=boolean  RndMeth=Simplest
  Resettable Delay : Delay  DelayLength=1  ExternalReset=Rising
      settings: InputPortMap=u0,r5
  Switch : Switch  Criteria=u2 ~= 0
  Switch1 : Switch  Criteria=u2 ~= 0
  Switch2 : Switch  Criteria=u2 ~= 0
  Terminator : Terminator
  Unit Delay : UnitDelay  SampleTime=-1
      settings: AttributesFormatString=InitialValue=%<InitialCondition>
  Unit Delay2 : UnitDelay  SampleTime=-1
      settings: AttributesFormatString=InitialValue=%<InitialCondition>
  EGRVlv_stJamVlv : Outport  Tag=%
  EGRVlv_bJamVlvRlsCheck_mp : Outport  Port=2
  wires:
  Logical Operator3/1 -> Debounce_DT/1
  EGRVlv_bGovDvtMinDeb_DSM/1 -> Logical Operator3/2
  EGRVlv_bGovDvtMaxDeb_DSM/1 -> Logical Operator3/1
  Constant16/1 -> Debounce_DT/4
  Relational Operator/1 -> Logical Operator/1
  CoEng_st/1 -> Relational Operator1/1
  Constant2/1 -> Relational Operator1/2
  Logical Operator/1 -> RSFilpFlop_Rp/2
  Constant3/1 -> Add1/1
  Debounce_DT/1 -> Logical Operator2/1, RSFilpFlop_Rp/1
  Relational Operator1/1 -> Detect Increase/1
  Detect Increase/1 -> Logical Operator/2
  Constant21/1 -> Product3/2
  Constant1/1 -> Product3/1
  Product3/1 -> Relational Operator/2
  Constant4/1 -> Product1/2
  Constant15/1 -> Product1/1
  Product1/1 -> Debounce_DT/2
  RSFilpFlop_Rp/2 -> Terminator/1
  Unit Delay/1 -> Switch/3, Add/2
  RSFilpFlop_Rp/1 -> Detect Increase1/1, Unit Delay2/1, Switch2/3  "EGRVlv_stJamVlv_mp"
  Detect Increase1/1 -> Switch/2
  Constant/1 -> Add/1
  Add/1 -> Switch/1
  Constant5/1 -> Relational Operator2/2
  Switch1/1 -> EGRVlv_stJamVlv/1, Switch2/1, Switch2/2
  Relational Operator2/1 -> Switch1/2
  Constant6/1 -> Switch1/1
  Constant7/1 -> Switch1/3
  [stJamVlv] -> Logical Operator1/1
  Unit Delay2/1 -> [stJamVlv]
  Switch2/1 -> EGRVlv_bJamVlvRlsCheck_mp/1  "EGRVlv_bJamVlvRlsCheck_mp"
  Switch/1 -> Relational Operator2/1, Unit Delay/1  "EGRVlv_numJamVlv_mp"
  Ground/1 -> Debounce_DT/3
  Logical Operator1/1 -> Logical Operator2/2
  Logical Operator2/1 -> Resettable Delay/2
  Add1/1 -> Resettable Delay/1, Relational Operator/1
  Resettable Delay/1 -> Add1/2

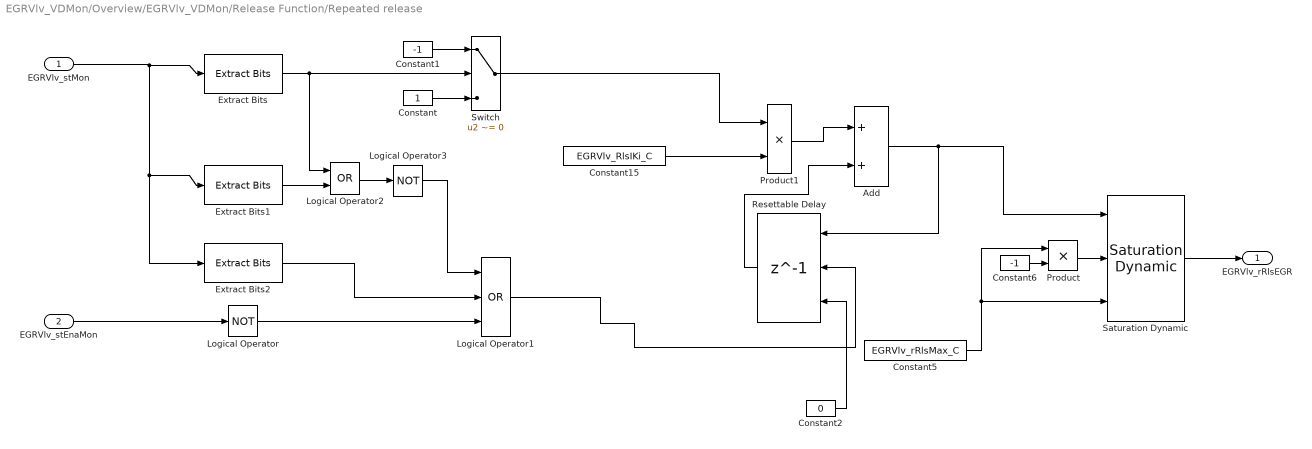
== system EGRVlv_VDMon/Overview/EGRVlv_VDMon/Release Function/Repeated release ==
  EGRVlv_stMon : Inport  Tag=%
  EGRVlv_stEnaMon : Inport  Tag=%  Port=2
  Add : Sum
  Constant : Constant  OutMin=-100  OutMax=100  OutDataTypeStr=DutyCycle
  Constant1 : Constant  Value=-1  OutMin=-100  OutMax=100  OutDataTypeStr=DutyCycle
  Constant15 : Constant  Value=EGRVlv_RlsIKi_C
  Constant2 : Constant  Value=0  OutDataTypeStr=DutyCycle
  Constant5 : Constant  Value=EGRVlv_rRlsMax_C
  Constant6 : Constant  Value=-1  OutDataTypeStr=int8
  Extract Bits : simulink/Logic and Bit Operations/Extract Bits  bitsToExtract=Range of bits  numBits=8  bitIdxRange=[8 8]  outScalingMode=Treat bit field as an integer
      settings: SourceProductName=Simulink
  Extract Bits1 : simulink/Logic and Bit Operations/Extract Bits  bitsToExtract=Range of bits  numBits=8  bitIdxRange=[6 6]  outScalingMode=Treat bit field as an integer
      settings: SourceProductName=Simulink
  Extract Bits2 : simulink/Logic and Bit Operations/Extract Bits  bitsToExtract=Range of bits  numBits=8  bitIdxRange=[10 10]  outScalingMode=Treat bit field as an integer
      settings: SourceProductName=Simulink
  Logical Operator : Logic  Operator=NOT  AllPortsSameDT=off  OutDataTypeStr=boolean
  Logical Operator1 : Logic  Operator=OR  Inputs=3  AllPortsSameDT=off  OutDataTypeStr=boolean
  Logical Operator2 : Logic  Operator=OR  AllPortsSameDT=off  OutDataTypeStr=boolean
  Logical Operator3 : Logic  Operator=NOT  AllPortsSameDT=off  OutDataTypeStr=boolean
  Product : Product  SaturateOnIntegerOverflow=on  OutDataTypeStr=Inherit: Same as first input
  Product1 : Product  OutDataTypeStr=Inherit: Same as first input
  Resettable Delay : Delay  DelayLength=1  InitialConditionSource=Input port  ExternalReset=Rising
      settings: InputPortMap=u0,r5,p4
  Saturation Dynamic : simulink/Discontinuities/Saturation Dynamic  OutMin=[]  OutMax=[]  OutDataTypeStr=Inherit: Same as second input  OutDataType=fixdt(1, 16)  OutScaling=2^-10  DoSatur=off
  Switch : Switch  Criteria=u2 ~= 0  InputSameDT=on
  EGRVlv_rRlsEGR : Outport  Tag=%
  wires:
  Product/1 -> Saturation Dynamic/2
  Logical Operator3/1 -> Logical Operator1/1
  Constant1/1 -> Switch/1
  Logical Operator/1 -> Logical Operator1/3
  Constant/1 -> Switch/3
  EGRVlv_stEnaMon/1 -> Logical Operator/1
  Extract Bits/1 -> Logical Operator2/1, Switch/2
  Switch/1 -> Product1/1
  Extract Bits1/1 -> Logical Operator2/2
  Logical Operator2/1 -> Logical Operator3/1
  Constant6/1 -> Product/2
  Extract Bits2/1 -> Logical Operator1/2
  Constant5/1 -> Saturation Dynamic/3, Product/1
  Add/1 -> Resettable Delay/1, Saturation Dynamic/1
  EGRVlv_stMon/1 -> Extract Bits/1, Extract Bits2/1, Extract Bits1/1
  Saturation Dynamic/1 -> EGRVlv_rRlsEGR/1
  Constant2/1 -> Resettable Delay/3
  Logical Operator1/1 -> Resettable Delay/2
  Constant15/1 -> Product1/2
  Product1/1 -> Add/1
  Resettable Delay/1 -> Add/2

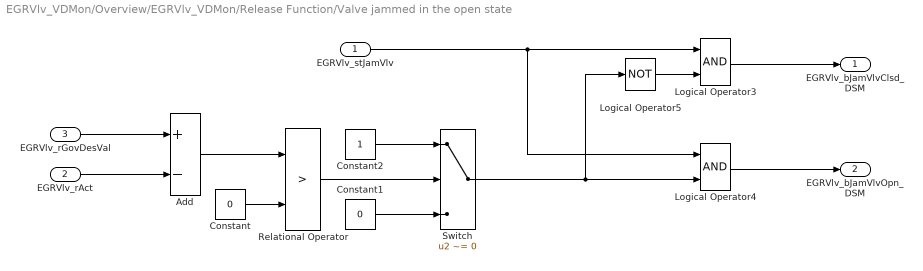
== system EGRVlv_VDMon/Overview/EGRVlv_VDMon/Release Function/Valve jammed in the open state ==
  EGRVlv_stJamVlv : Inport  Tag=%
  EGRVlv_rAct : Inport  Tag=%  Port=2
  EGRVlv_rGovDesVal : Inport  Tag=%  Port=3
  Add : Sum  Inputs=+-
  Constant : Constant  Value=0  OutDataTypeStr=Inherit: Inherit via back propagation
  Constant1 : Constant  Value=0  OutDataTypeStr=boolean
  Constant2 : Constant  OutDataTypeStr=boolean
  Logical Operator3 : Logic  AllPortsSameDT=off  OutDataTypeStr=boolean
  Logical Operator4 : Logic  AllPortsSameDT=off  OutDataTypeStr=boolean
  Logical Operator5 : Logic  Operator=NOT  AllPortsSameDT=off  OutDataTypeStr=boolean
  Relational Operator : RelationalOperator  Operator=>  OutDataTypeStr=boolean  RndMeth=Simplest  InputSameDT=on
  Switch : Switch  Criteria=u2 ~= 0
  EGRVlv_bJamVlvClsd_DSM : Outport  Tag=%
  EGRVlv_bJamVlvOpn_DSM : Outport  Tag=%  Port=2
  wires:
  Switch/1 -> Logical Operator5/1, Logical Operator4/2
  Logical Operator3/1 -> EGRVlv_bJamVlvClsd_DSM/1
  Logical Operator5/1 -> Logical Operator3/2
  Logical Operator4/1 -> EGRVlv_bJamVlvOpn_DSM/1
  EGRVlv_stJamVlv/1 -> Logical Operator4/1, Logical Operator3/1
  EGRVlv_rGovDesVal/1 -> Add/1
  EGRVlv_rAct/1 -> Add/2
  Add/1 -> Relational Operator/1
  Constant/1 -> Relational Operator/2
  Relational Operator/1 -> Switch/2
  Constant1/1 -> Switch/3
  Constant2/1 -> Switch/1
